simulink library "SUB_ECU_L4_MABX_HW_Interface_PTC_166"  (R2018a)
settings: Solver=VariableStepAuto  StartTime=0.0  StopTime=10.0  RelTol=1e-3
PostLoadFcn:
  | , if any(exist('dsrtsu_mdlpostloadfcn', 'file') == [2, 3, 6]), try dsrtsu_mdlpostloadfcn('Execute', bdroot); catch fprintf('Error in PostLoadFcn (dsrtsu_mdlpostloadfcn) for model "%s":\n %s\n', bdroot, lasterr); end, end,
undefined symbols (not defined in the file or in its folder): CANR_PROPB_REAX_3_13_CHANNEL_APV, CANR_PROPB_REAX_4_13_CHANNEL_APV, CANR_PROPB_XPR_1_50_CHANNEL_APV, ENUM_CAN_RX_T, ENUM_CAN_TX_T, ENUM_REAX_OPERATION_MODE_T, ENUM_SIGNAL_HEALTH_T, ENUM_XBR_CONTROL_MODE_T, ENUM_XBR_EBI_MODE_T, ENUM_XBR_PASS_THROUGH_ACTIVE_T, ENUM_XBR_PRIORITY_T, ENUM_XPR_INHIBIT_PARK_MANUAL_T, ENUM_XPR_INHIBIT_UNPARK_MANUAL_T, ENUM_XPR_PARK_MANUAL_T, ENUM_XPR_UNPARK_MANUAL_T, PROPB_REAX_1_E4_DES_POS_SIG_SRC_APV, PROPB_REAX_1_E4_DESIRED_OPMODE_APV, PROPB_REAX_1_E4_DESIRED_POSITION_APV, ptc_matlab_lib
libraries: PTC_MBDS_LIB x163, rtican x79, simulink x41, EmE_MBD_Blockset x35, rti1401lib_dio_type4 x8, simulink_need_slupdate x7, $bdroot x5, rti1401lib_adc_type4 x3, rtitasklib x1
(part 3 of 25)

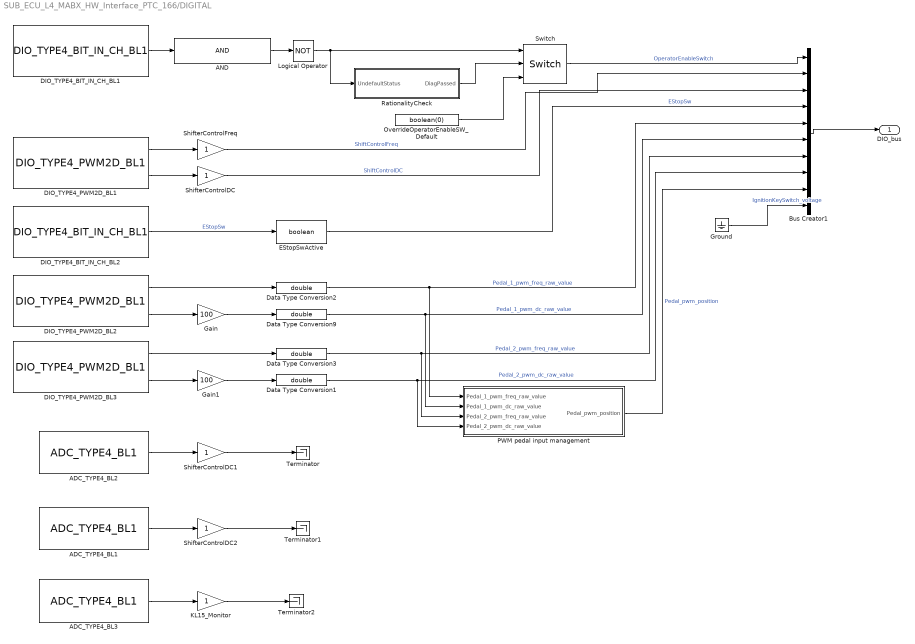
== system SUB_ECU_L4_MABX_HW_Interface_PTC_166/DIGITAL ==
  ADC_TYPE4_BL1 : rti1401lib_adc_type4/ADC_TYPE4_BL1  DSProperties=struct('RTI',struct('Version',uint32(2),'BlockType',struct('isSLSource',uint8(1),'isSLSink',uint8(1),'isHWSource',uint8(0),'isHWSink',uint8(1),'isSetup',uint8(0),'isInline',uint8(1),'isNonInline',uint8(0),'isInterrupt',uint8(0),'isChannelwise',uint8(1)),'IOBoardType',{{'DS1401','STD','ADCT4'}},'UnitType','ADC','Identifier','ADC','DialogType','ML','BlockSet','NONE','SlaveProcessor','NONE'))  RTIBlockInterface=struct('InputPortsActive',0,'InputPortsWidth',int32(1),'InputPortsDataType',{{'SS_BOOLEAN'}},'InputPortsName',{{'Continue'}},'OutputPortsActive',[1 0],'OutputPortsWidth',int32([1 1]),'OutputPortsDataType',{{'SS_DOUBLE','SS_UINT8'}},'OutputPortsName',{{'ADC','Status'}},'DialogFcn','rti1401stdadct4adcgui','SampleTime',{{-1}},'InitLevel',3,'IconTransparency','on','BlockDisplay',{{['ADC TP4\nModule: 1\nChannel: 2'],'center'}},'BlockName',struct('Token',{{'ADC_TYPE4_BL1'}}))  RTIBlockParameters=struct('ADCSWStartDisable',{{0,'OFF',[0 1]}},'ModuleNo',{{1,'OFF',[1 16]}},'ChannelNo',{{2,'OFF',[1 16]}},'ConversionMode',{{1,'OFF',[1 2]}},'SampleMode',{{1,'OFF',[1 2]}},'TriggerSource',{{1,'OFF',[1 5]}},'EdgePolarity',{{1,'OFF',[1 2]}},'ConversionTriggerSource',{{2,'OFF',[1 6]}},'ConversionEdgePolarity',{{1,'OFF',[1 2]}},'ConversionPeriod',{{'1e-06','OFF',[]}},'ConversionPeriodCheck',{{0,'OFF',[]}},'BurstTriggerSource',{{1,'OFF',[1 6]}},'BurstEdgePolarity',{{1,'OFF',[1 2]}},'BurstSize',{{'10','OFF',[]}},'BurstSizeCheck',{{0,'OFF',[]}},'DataSetOffset',{{'0','OFF',[]}},'DataSetOffsetCheck',{{0,'OFF',[]}},'DataSetLength',{{'1','OFF',[]}},'DataSetLengthCheck',{{0,'OFF',[]}},'ReadMode',{{1,'OFF',[1 2]}},'SampleTime',{{'-1','OFF',[-1 inf]}},'SampleTimeCheck',{{1,'OFF',[]}},'StatusPortEnable',{{0,'OFF',[0 1]}},'VoltageRange',{{2,'OFF',[1 2]}},'TLCFileName',{{'rti1401adc_t4_adc','OFF',[]}})  RTISFcnParameters=struct('ADCSWStartDisable','int32','ModuleNo','int32','ChannelNo','int16','ConversionMode','int16','SampleMode','int16','TriggerSource','int16','EdgePolarity','int16','ConversionTriggerSource','int16','ConversionEdgePolarity','int16','ConversionPeriod','double','BurstTriggerSource','int16','BurstEdgePolarity','int16','BurstSize','int16','DataSetOffset','int16','DataSetLength','int16','ReadMode','int16','SampleTime','double','StatusPortEnable','int16','VoltageRange','int16','TLCFileName','char')  RTIBlockParaDefault=struct('ADCSWStartDisable',0,'ModuleNo',1,'ChannelNo',1,'ConversionMode',1,'SampleMode',1,'TriggerSource',1,'EdgePolarity',1,'ConversionTriggerSource',2,'ConversionEdgePolarity',1,'ConversionPeriod',1e-6,'ConversionPeriodCheck',0,'BurstTriggerSource',1,'BurstEdgePolarity',1,'BurstSize',10,'BurstSizeCheck',0,'DataSetOffset',0,'DataSetOffsetCheck',0,'DataSetLength',1,'DataSetLengthCheck',0,'ReadMode',1,'SampleTime',-1,'SampleTimeCheck',1,'StatusPortEnable',0,'VoltageRange',1,'TLCFileName','rti1401adc_t4_adc')
  ADC_TYPE4_BL2 : rti1401lib_adc_type4/ADC_TYPE4_BL1  DSProperties=struct('RTI',struct('Version',uint32(2),'BlockType',struct('isSLSource',uint8(1),'isSLSink',uint8(1),'isHWSource',uint8(0),'isHWSink',uint8(1),'isSetup',uint8(0),'isInline',uint8(1),'isNonInline',uint8(0),'isInterrupt',uint8(0),'isChannelwise',uint8(1)),'IOBoardType',{{'DS1401','STD','ADCT4'}},'UnitType','ADC','Identifier','ADC','DialogType','ML','BlockSet','NONE','SlaveProcessor','NONE'))  RTIBlockInterface=struct('InputPortsActive',0,'InputPortsWidth',int32(1),'InputPortsDataType',{{'SS_BOOLEAN'}},'InputPortsName',{{'Continue'}},'OutputPortsActive',[1 0],'OutputPortsWidth',int32([1 1]),'OutputPortsDataType',{{'SS_DOUBLE','SS_UINT8'}},'OutputPortsName',{{'ADC','Status'}},'DialogFcn','rti1401stdadct4adcgui','SampleTime',{{-1}},'InitLevel',3,'IconTransparency','on','BlockDisplay',{{['ADC TP4\nModule: 1\nChannel: 1'],'center'}},'BlockName',struct('Token',{{'ADC_TYPE4_BL1'}}))  RTIBlockParameters=struct('ADCSWStartDisable',{{0,'OFF',[0 1]}},'ModuleNo',{{1,'OFF',[1 16]}},'ChannelNo',{{1,'OFF',[1 16]}},'ConversionMode',{{1,'OFF',[1 2]}},'SampleMode',{{1,'OFF',[1 2]}},'TriggerSource',{{1,'OFF',[1 5]}},'EdgePolarity',{{1,'OFF',[1 2]}},'ConversionTriggerSource',{{2,'OFF',[1 6]}},'ConversionEdgePolarity',{{1,'OFF',[1 2]}},'ConversionPeriod',{{'1e-06','OFF',[]}},'ConversionPeriodCheck',{{0,'OFF',[]}},'BurstTriggerSource',{{1,'OFF',[1 6]}},'BurstEdgePolarity',{{1,'OFF',[1 2]}},'BurstSize',{{'10','OFF',[]}},'BurstSizeCheck',{{0,'OFF',[]}},'DataSetOffset',{{'0','OFF',[]}},'DataSetOffsetCheck',{{0,'OFF',[]}},'DataSetLength',{{'1','OFF',[]}},'DataSetLengthCheck',{{0,'OFF',[]}},'ReadMode',{{1,'OFF',[1 2]}},'SampleTime',{{'-1','OFF',[-1 inf]}},'SampleTimeCheck',{{1,'OFF',[]}},'StatusPortEnable',{{0,'OFF',[0 1]}},'VoltageRange',{{2,'OFF',[1 2]}},'TLCFileName',{{'rti1401adc_t4_adc','OFF',[]}})  RTISFcnParameters=struct('ADCSWStartDisable','int32','ModuleNo','int32','ChannelNo','int16','ConversionMode','int16','SampleMode','int16','TriggerSource','int16','EdgePolarity','int16','ConversionTriggerSource','int16','ConversionEdgePolarity','int16','ConversionPeriod','double','BurstTriggerSource','int16','BurstEdgePolarity','int16','BurstSize','int16','DataSetOffset','int16','DataSetLength','int16','ReadMode','int16','SampleTime','double','StatusPortEnable','int16','VoltageRange','int16','TLCFileName','char')  RTIBlockParaDefault=struct('ADCSWStartDisable',0,'ModuleNo',1,'ChannelNo',1,'ConversionMode',1,'SampleMode',1,'TriggerSource',1,'EdgePolarity',1,'ConversionTriggerSource',2,'ConversionEdgePolarity',1,'ConversionPeriod',1e-6,'ConversionPeriodCheck',0,'BurstTriggerSource',1,'BurstEdgePolarity',1,'BurstSize',10,'BurstSizeCheck',0,'DataSetOffset',0,'DataSetOffsetCheck',0,'DataSetLength',1,'DataSetLengthCheck',0,'ReadMode',1,'SampleTime',-1,'SampleTimeCheck',1,'StatusPortEnable',0,'VoltageRange',1,'TLCFileName','rti1401adc_t4_adc')
  ADC_TYPE4_BL3 : rti1401lib_adc_type4/ADC_TYPE4_BL1  DSProperties=struct('RTI',struct('Version',uint32(2),'BlockType',struct('isSLSource',uint8(1),'isSLSink',uint8(1),'isHWSource',uint8(0),'isHWSink',uint8(1),'isSetup',uint8(0),'isInline',uint8(1),'isNonInline',uint8(0),'isInterrupt',uint8(0),'isChannelwise',uint8(1)),'IOBoardType',{{'DS1401','STD','ADCT4'}},'UnitType','ADC','Identifier','ADC','DialogType','ML','BlockSet','NONE','SlaveProcessor','NONE'))  RTIBlockInterface=struct('InputPortsActive',0,'InputPortsWidth',int32(1),'InputPortsDataType',{{'SS_BOOLEAN'}},'InputPortsName',{{'Continue'}},'OutputPortsActive',[1 0],'OutputPortsWidth',int32([1 1]),'OutputPortsDataType',{{'SS_DOUBLE','SS_UINT8'}},'OutputPortsName',{{'ADC','Status'}},'DialogFcn','rti1401stdadct4adcgui','SampleTime',{{-1}},'InitLevel',3,'IconTransparency','on','BlockDisplay',{{['ADC TP4\nModule: 1\nChannel: 3'],'center'}},'BlockName',struct('Token',{{'ADC_TYPE4_BL1'}}))  RTIBlockParameters=struct('ADCSWStartDisable',{{0,'OFF',[0 1]}},'ModuleNo',{{1,'OFF',[1 16]}},'ChannelNo',{{3,'OFF',[1 16]}},'ConversionMode',{{1,'OFF',[1 2]}},'SampleMode',{{1,'OFF',[1 2]}},'TriggerSource',{{1,'OFF',[1 5]}},'EdgePolarity',{{1,'OFF',[1 2]}},'ConversionTriggerSource',{{2,'OFF',[1 6]}},'ConversionEdgePolarity',{{1,'OFF',[1 2]}},'ConversionPeriod',{{'1e-06','OFF',[]}},'ConversionPeriodCheck',{{0,'OFF',[]}},'BurstTriggerSource',{{1,'OFF',[1 6]}},'BurstEdgePolarity',{{1,'OFF',[1 2]}},'BurstSize',{{'10','OFF',[]}},'BurstSizeCheck',{{0,'OFF',[]}},'DataSetOffset',{{'0','OFF',[]}},'DataSetOffsetCheck',{{0,'OFF',[]}},'DataSetLength',{{'1','OFF',[]}},'DataSetLengthCheck',{{0,'OFF',[]}},'ReadMode',{{1,'OFF',[1 2]}},'SampleTime',{{'-1','OFF',[-1 inf]}},'SampleTimeCheck',{{1,'OFF',[]}},'StatusPortEnable',{{0,'OFF',[0 1]}},'VoltageRange',{{2,'OFF',[1 2]}},'TLCFileName',{{'rti1401adc_t4_adc','OFF',[]}})  RTISFcnParameters=struct('ADCSWStartDisable','int32','ModuleNo','int32','ChannelNo','int16','ConversionMode','int16','SampleMode','int16','TriggerSource','int16','EdgePolarity','int16','ConversionTriggerSource','int16','ConversionEdgePolarity','int16','ConversionPeriod','double','BurstTriggerSource','int16','BurstEdgePolarity','int16','BurstSize','int16','DataSetOffset','int16','DataSetLength','int16','ReadMode','int16','SampleTime','double','StatusPortEnable','int16','VoltageRange','int16','TLCFileName','char')  RTIBlockParaDefault=struct('ADCSWStartDisable',0,'ModuleNo',1,'ChannelNo',1,'ConversionMode',1,'SampleMode',1,'TriggerSource',1,'EdgePolarity',1,'ConversionTriggerSource',2,'ConversionEdgePolarity',1,'ConversionPeriod',1e-6,'ConversionPeriodCheck',0,'BurstTriggerSource',1,'BurstEdgePolarity',1,'BurstSize',10,'BurstSizeCheck',0,'DataSetOffset',0,'DataSetOffsetCheck',0,'DataSetLength',1,'DataSetLengthCheck',0,'ReadMode',1,'SampleTime',-1,'SampleTimeCheck',1,'StatusPortEnable',0,'VoltageRange',1,'TLCFileName','rti1401adc_t4_adc')
  AND : PTC_MBDS_LIB/MBDS Standard Library/Basic Operations/Logic and Bit Operations/AND  BitwiseMode=on  Inputs=1  UseBitMask=on  BitMask=bin2dec('0000000000000001')  OutDataTypeStr=boolean  PTC_MBDS_BlockVersion=5.41  PTC_BlockType=PTC_MBDS_AND
      settings: AttributesFormatString=bitwise  SourceProductName=PACCAR Technical Center MBDS Library
  Bus Creator1 : BusCreator  Inputs=10
  DIO_TYPE4_BIT_IN_CH_BL1 : rti1401lib_dio_type4/DIO_TYPE4_BIT_IN_CH_BL1  DSProperties=struct('RTI',struct('Version',uint32(1),'BlockType',struct('isSLSource',uint8(1),'isSLSink',uint8(0),'isHWSource',uint8(1),'isHWSink',uint8(0),'isSetup',uint8(0),'isInline',uint8(1),'isNonInline',uint8(0),'isInterrupt',uint8(0),'isChannelwise',uint8(1)),'IOBoardType',{{'DS1401','STD','DIOT4'}},'UnitType','BIT','Identifier','BITINCH','DialogType','ML','BlockSet','NONE','SlaveProcessor','NONE'))  RTIBlockInterface=struct('OutputPortsWidth',int32(1),'OutputPortsDataType',{{'SS_BOOLEAN'}},'OutputPortsActive',1,'OutputPortsName',{{'Out'}},'BlockDisplay',{{['DIO TP4 BIT IN\n Channelwise\nModule: 1\nPort: 1\nChannel: 1'],'center'}},'IconTransparency','on','InitLevel',3,'DialogFcn','rti1401stddiot4bitinchgui','BlockName',struct('Token',{{'DIO_TYPE4_BIT_IN_CH_BL1'}}))  RTIBlockParameters=struct('ModuleNo',{{1,'OFF',[1 16]}},'PortNo',{{1,'OFF',[1 2]}},'ChannelNo',{{1,'OFF',[1 16]}},'TLCFileName',{{'rti1401dio_t4_bit_in_ch','OFF',[]}},'EnableInterrupt',{{0,'OFF',[0 1]}},'TriggerEdgeType',{{1,'OFF',[1 3]}})  RTISFcnParameters=struct('ModuleNo','int32','PortNo','int16','ChannelNo','int16','TLCFileName','char','EnableInterrupt','int16','TriggerEdgeType','int32')  RTIBlockParaDefault=struct('ModuleNo',1,'PortNo',1,'ChannelNo',1,'TLCFileName','rti1401dio_t4_bit_in_ch','EnableInterrupt',0,'TriggerEdgeType',1)
  DIO_TYPE4_BIT_IN_CH_BL2 : rti1401lib_dio_type4/DIO_TYPE4_BIT_IN_CH_BL1  DSProperties=struct('RTI',struct('Version',uint32(1),'BlockType',struct('isSLSource',uint8(1),'isSLSink',uint8(0),'isHWSource',uint8(1),'isHWSink',uint8(0),'isSetup',uint8(0),'isInline',uint8(1),'isNonInline',uint8(0),'isInterrupt',uint8(0),'isChannelwise',uint8(1)),'IOBoardType',{{'DS1401','STD','DIOT4'}},'UnitType','BIT','Identifier','BITINCH','DialogType','ML','BlockSet','NONE','SlaveProcessor','NONE'))  RTIBlockInterface=struct('OutputPortsWidth',int32(1),'OutputPortsDataType',{{'SS_BOOLEAN'}},'OutputPortsActive',1,'OutputPortsName',{{'Out'}},'BlockDisplay',{{['DIO TP4 BIT IN\n Channelwise\nModule: 1\nPort: 1\nChannel: 3'],'center'}},'IconTransparency','on','InitLevel',3,'DialogFcn','rti1401stddiot4bitinchgui','BlockName',struct('Token',{{'DIO_TYPE4_BIT_IN_CH_BL1'}}))  RTIBlockParameters=struct('ModuleNo',{{1,'OFF',[1 16]}},'PortNo',{{1,'OFF',[1 2]}},'ChannelNo',{{3,'OFF',[1 16]}},'TLCFileName',{{'rti1401dio_t4_bit_in_ch','OFF',[]}},'EnableInterrupt',{{0,'OFF',[0 1]}},'TriggerEdgeType',{{1,'OFF',[1 3]}})  RTISFcnParameters=struct('ModuleNo','int32','PortNo','int16','ChannelNo','int16','TLCFileName','char','EnableInterrupt','int16','TriggerEdgeType','int32')  RTIBlockParaDefault=struct('ModuleNo',1,'PortNo',1,'ChannelNo',1,'TLCFileName','rti1401dio_t4_bit_in_ch','EnableInterrupt',0,'TriggerEdgeType',1)
  DIO_TYPE4_PWM2D_BL1 : rti1401lib_dio_type4/DIO_TYPE4_PWM2D_BL1  DSProperties=struct('RTI',struct('Version',uint32(1),'BlockType',struct('isSLSource',uint8(1),'isSLSink',uint8(0),'isHWSource',uint8(1),'isHWSink',uint8(0),'isSetup',uint8(0),'isInline',uint8(1),'isNonInline',uint8(0),'isInterrupt',uint8(0),'isChannelwise',uint8(1)),'IOBoardType',{{'DS1401','STD','DIOT4'}},'UnitType','PWM','Identifier','PWM2D','DialogType','ML','BlockSet','NONE','SlaveProcessor','NONE'))  RTIBlockInterface=struct('OutputPortsWidth',int32([1 1]),'OutputPortsActive',[1 1],'OutputPortsName',{{'Frequency',['Duty Cycle']}},'BlockDisplay',{{['DIO TP4 PWM2D\nModule: 1\nPort: 1\nChannel: 2'],'center'}},'IconTransparency','on','InitLevel',3,'DialogFcn','rti1401stddiot4pwm2dgui','BlockName',struct('Token',{{'DIO_TYPE4_PWM2D_BL1'}}))  RTIBlockParameters=struct('ModuleNo',{{1,'ON',[1 16]}},'PortNo',{{1,'OFF',[1 2]}},'ChannelNo',{{2,'ON',[1 16]}},'UpdateMode',{{1,'ON',[1 2]}},'FrequencyRange',{{7,'OFF',[1 16]}},'TLCFileName',{{'rti1401dio_t4_pwm2d','OFF',[]}},'EnableInterrupt',{{0,'OFF',[0 1]}},'TriggerEdgeType',{{1,'OFF',[1 3]}})  RTISFcnParameters=struct('ModuleNo','int32','PortNo','int16','ChannelNo','int16','UpdateMode','int16','FrequencyRange','int16','TLCFileName','char','EnableInterrupt','int16','TriggerEdgeType','int32')  RTIBlockParaDefault=struct('ModuleNo',1,'PortNo',1,'ChannelNo',1,'UpdateMode',1,'FrequencyRange',7,'TLCFileName','rti1401dio_t4_pwm2d','EnableInterrupt',0,'TriggerEdgeType',1)
  DIO_TYPE4_PWM2D_BL2 : rti1401lib_dio_type4/DIO_TYPE4_PWM2D_BL1  DSProperties=struct('RTI',struct('Version',uint32(1),'BlockType',struct('isSLSource',uint8(1),'isSLSink',uint8(0),'isHWSource',uint8(1),'isHWSink',uint8(0),'isSetup',uint8(0),'isInline',uint8(1),'isNonInline',uint8(0),'isInterrupt',uint8(0),'isChannelwise',uint8(1)),'IOBoardType',{{'DS1401','STD','DIOT4'}},'UnitType','PWM','Identifier','PWM2D','DialogType','ML','BlockSet','NONE','SlaveProcessor','NONE'))  RTIBlockInterface=struct('OutputPortsWidth',int32([1 1]),'OutputPortsActive',[1 1],'OutputPortsName',{{'Frequency',['Duty Cycle']}},'BlockDisplay',{{['DIO TP4 PWM2D\nModule: 1\nPort: 2\nChannel: 1'],'center'}},'IconTransparency','on','InitLevel',3,'DialogFcn','rti1401stddiot4pwm2dgui','BlockName',struct('Token',{{'DIO_TYPE4_PWM2D_BL1'}}))  RTIBlockParameters=struct('ModuleNo',{{1,'ON',[1 16]}},'PortNo',{{2,'OFF',[1 2]}},'ChannelNo',{{1,'ON',[1 8]}},'UpdateMode',{{1,'ON',[1 2]}},'FrequencyRange',{{12,'OFF',[1 16]}},'TLCFileName',{{'rti1401dio_t4_pwm2d','OFF',[]}},'EnableInterrupt',{{0,'OFF',[0 1]}},'TriggerEdgeType',{{1,'OFF',[1 3]}})  RTISFcnParameters=struct('ModuleNo','int32','PortNo','int16','ChannelNo','int16','UpdateMode','int16','FrequencyRange','int16','TLCFileName','char','EnableInterrupt','int16','TriggerEdgeType','int32')  RTIBlockParaDefault=struct('ModuleNo',1,'PortNo',1,'ChannelNo',1,'UpdateMode',1,'FrequencyRange',7,'TLCFileName','rti1401dio_t4_pwm2d','EnableInterrupt',0,'TriggerEdgeType',1)
  DIO_TYPE4_PWM2D_BL3 : rti1401lib_dio_type4/DIO_TYPE4_PWM2D_BL1  DSProperties=struct('RTI',struct('Version',uint32(1),'BlockType',struct('isSLSource',uint8(1),'isSLSink',uint8(0),'isHWSource',uint8(1),'isHWSink',uint8(0),'isSetup',uint8(0),'isInline',uint8(1),'isNonInline',uint8(0),'isInterrupt',uint8(0),'isChannelwise',uint8(1)),'IOBoardType',{{'DS1401','STD','DIOT4'}},'UnitType','PWM','Identifier','PWM2D','DialogType','ML','BlockSet','NONE','SlaveProcessor','NONE'))  RTIBlockInterface=struct('OutputPortsWidth',int32([1 1]),'OutputPortsActive',[1 1],'OutputPortsName',{{'Frequency',['Duty Cycle']}},'BlockDisplay',{{['DIO TP4 PWM2D\nModule: 1\nPort: 2\nChannel: 2'],'center'}},'IconTransparency','on','InitLevel',3,'DialogFcn','rti1401stddiot4pwm2dgui','BlockName',struct('Token',{{'DIO_TYPE4_PWM2D_BL1'}}))  RTIBlockParameters=struct('ModuleNo',{{1,'ON',[1 16]}},'PortNo',{{2,'OFF',[1 2]}},'ChannelNo',{{2,'ON',[1 8]}},'UpdateMode',{{1,'ON',[1 2]}},'FrequencyRange',{{12,'OFF',[1 16]}},'TLCFileName',{{'rti1401dio_t4_pwm2d','OFF',[]}},'EnableInterrupt',{{0,'OFF',[0 1]}},'TriggerEdgeType',{{1,'OFF',[1 3]}})  RTISFcnParameters=struct('ModuleNo','int32','PortNo','int16','ChannelNo','int16','UpdateMode','int16','FrequencyRange','int16','TLCFileName','char','EnableInterrupt','int16','TriggerEdgeType','int32')  RTIBlockParaDefault=struct('ModuleNo',1,'PortNo',1,'ChannelNo',1,'UpdateMode',1,'FrequencyRange',7,'TLCFileName','rti1401dio_t4_pwm2d','EnableInterrupt',0,'TriggerEdgeType',1)
  Data Type Conversion{1..3,9} (4 alike) : DataTypeConversion  OutDataTypeStr=double  SaturateOnIntegerOverflow=on
  EStopSwActive : DataTypeConversion  OutDataTypeStr=boolean
  Gain : Gain  Gain=100
  Gain1 : Gain  Gain=100
  Ground : Ground
  KL15_Monitor : Gain
  Logical Operator : Logic  Operator=NOT  AllPortsSameDT=off  OutDataTypeStr=boolean
  OverrideOperatorEnableSW_Default : Constant  Value=boolean(0)
  PWM pedal input management : Subsystem
  RationalityCheck : Subsystem
  ShifterControlDC : Gain
  ShifterControlDC1 : Gain
  ShifterControlDC2 : Gain
  ShifterControlFreq : Gain
  Switch : PTC_MBDS_LIB/MBDS Standard Library/Signals & Systems/Signal Routing/Switch  OutDataTypeStr_=Inherit: Inherit via back propagation  SaturateOnIntegerOverflow_=on  InputSameDT_=on  PTC_MBDS_BlockVersion=5.41  PTC_BlockType=PTC_MBDS_Switch
      settings: SourceProductName=PACCAR Technical Center MBDS Library
  Terminator : Terminator
  Terminator1 : Terminator
  Terminator2 : Terminator
  DIO_bus : Outport
  wires:
  ShifterControlDC2/1 -> Terminator1/1
  ShifterControlDC1/1 -> Terminator/1
  ADC_TYPE4_BL2/1 -> ShifterControlDC1/1
  ADC_TYPE4_BL1/1 -> ShifterControlDC2/1
  Data Type Conversion1/1 -> PWM pedal input management/4(Pedal_2_pwm_dc_raw_value), Bus Creator1/8  "Pedal_2_pwm_dc_raw_value"
  Data Type Conversion3/1 -> PWM pedal input management/3(Pedal_2_pwm_freq_raw_value), Bus Creator1/7  "Pedal_2_pwm_freq_raw_value"
  Data Type Conversion9/1 -> PWM pedal input management/2(Pedal_1_pwm_dc_raw_value), Bus Creator1/6  "Pedal_1_pwm_dc_raw_value"
  Data Type Conversion2/1 -> PWM pedal input management/1(Pedal_1_pwm_freq_raw_value), Bus Creator1/5  "Pedal_1_pwm_freq_raw_value"
  PWM pedal input management/1(Pedal_pwm_position) -> Bus Creator1/9  "Pedal_pwm_position"
  Gain1/1 -> Data Type Conversion1/1
  Gain/1 -> Data Type Conversion9/1
  DIO_TYPE4_PWM2D_BL3/1 -> Data Type Conversion3/1
  DIO_TYPE4_PWM2D_BL2/1 -> Data Type Conversion2/1
  DIO_TYPE4_PWM2D_BL3/2 -> Gain1/1
  DIO_TYPE4_PWM2D_BL2/2 -> Gain/1
  DIO_TYPE4_BIT_IN_CH_BL1/1 -> AND/1
  Switch/1 -> Bus Creator1/1  "OperatorEnableSwitch"
  AND/1 -> Logical Operator/1
  DIO_TYPE4_PWM2D_BL1/1 -> ShifterControlFreq/1
  DIO_TYPE4_PWM2D_BL1/2 -> ShifterControlDC/1
  Bus Creator1/1 -> DIO_bus/1
  ShifterControlFreq/1 -> Bus Creator1/2  "ShiftControlFreq"
  ShifterControlDC/1 -> Bus Creator1/3  "ShiftControlDC"
  EStopSwActive/1 -> Bus Creator1/4  "EStopSw"
  Logical Operator/1 -> RationalityCheck/1(UndefaultStatus), Switch/1
  OverrideOperatorEnableSW_Default/1 -> Switch/3
  RationalityCheck/1(DiagPassed) -> Switch/2
  DIO_TYPE4_BIT_IN_CH_BL2/1 -> EStopSwActive/1  "EStopSw"
  ADC_TYPE4_BL3/1 -> KL15_Monitor/1
  KL15_Monitor/1 -> Terminator2/1
  Ground/1 -> Bus Creator1/10  "IgnitionKeySwitch_voltage"

== system SUB_ECU_L4_MABX_HW_Interface_PTC_166/DIGITAL_out ==
  Out : Inport
  In : Inport  Port=2
  Bus Selector : BusSelector  OutputSignals=10msTask.APTC.APTC_arb_pedal_position
  Constant1 : Constant
  Constant2 : Constant  Value=0.001
  Constant3 : Constant
  Constant4 : Constant  Value=0.001
  DIO_TYPE4_BIT_OUT_CH_BL1 : rti1401lib_dio_type4/DIO_TYPE4_BIT_OUT_CH_BL1  DSProperties=struct('RTI',struct('Version',uint32(1),'BlockType',struct('isSLSource',uint8(0),'isSLSink',uint8(1),'isHWSource',uint8(0),'isHWSink',uint8(1),'isSetup',uint8(0),'isInline',uint8(1),'isNonInline',uint8(0),'isInterrupt',uint8(0),'isChannelwise',uint8(1)),'IOBoardType',{{'DS1401','STD','DIOT4'}},'UnitType','BIT','Identifier','BITOUTCH','DialogType','ML','BlockSet','NONE','SlaveProcessor','NONE'))  RTIBlockInterface=struct('InputPortsWidth',int32(1),'InputPortsActive',1,'InputPortsDataType',{{'SS_BOOLEAN'}},'InputPortsName',{{'In'}},'BlockDisplay',{{['DIO TP4 BIT OUT\n Channelwise\nModule: 1\nPort: 1\nChannel: 3'],'center'}},'IconTransparency','on','InitLevel',3,'DialogFcn','rti1401stddiot4bitoutchgui','BlockName',struct('Token',{{'DIO_TYPE4_BIT_OUT_CH_BL1'}}))  RTIBlockParameters=struct('ModuleNo',{{1,'OFF',[1 16]}},'PortNo',{{1,'OFF',[1 2]}},'ChannelNo',{{3,'OFF',[1 16]}},'OutputStateInit',{{0,'OFF',[0 1]}},'TerminationMode',{{0,'OFF',[0 1]}},'OutputStateTermValidate',{{0,'OFF',[0 1]}},'OutputStateTerm',{{0,'OFF',[0 1]}},'SupplyRailsCh',{{[1 0],'OFF',[0 1 0 1]}},'TLCFileName',{{'rti1401dio_t4_bit_out_ch','OFF',[]}},'EnableInterrupt',{{0,'OFF',[0 1]}},'TriggerEdgeType',{{1,'OFF',[1 3]}})  RTISFcnParameters=struct('ModuleNo','int32','PortNo','int16','ChannelNo','int16','SupplyRailsCh','int16','OutputStateInit','int16','TerminationMode','int16','OutputStateTermValidate','int16','OutputStateTerm','int16','TLCFileName','char','EnableInterrupt','int16','TriggerEdgeType','int32')  RTIBlockParaDefault=struct('ModuleNo',1,'PortNo',1,'ChannelNo',1,'OutputStateInit',0,'TerminationMode',0,'OutputStateTermValidate',0,'OutputStateTerm',0,'SupplyRailsCh',[1 1],'TLCFileName','rti1401dio_t4_bit_out_ch','EnableInterrupt',0,'TriggerEdgeType',1)
  DIO_TYPE4_PWM_BL1 : rti1401lib_dio_type4/DIO_TYPE4_PWM_BL1  DSProperties=struct('RTI',struct('Version',uint32(1),'BlockType',struct('isSLSource',uint8(0),'isSLSink',uint8(1),'isHWSource',uint8(0),'isHWSink',uint8(1),'isSetup',uint8(0),'isInline',uint8(1),'isNonInline',uint8(0),'isInterrupt',uint8(0),'isChannelwise',uint8(1)),'IOBoardType',{{'DS1401','STD','DIOT4'}},'UnitType','PWM','Identifier','PWM','DialogType','ML','BlockSet','NONE','SlaveProcessor','NONE'))  RTIBlockInterface=struct('InputPortsWidth',int32([1 1]),'InputPortsActive',[1 1],'InputPortsName',{{'Period',['Duty Cycle']}},'BlockDisplay',{{['DIO TP4 PWM\nModule: 1\nPort: 2\nChannel: 1'],'center'}},'IconTransparency','on','InitLevel',3,'DialogFcn','rti1401stddiot4pwmgui','BlockName',struct('Token',{{'DIO_TYPE4_PWM_BL1'}}))  RTIBlockParameters=struct('ModuleNo',{{1,'OFF',[1 16]}},'PortNo',{{2,'OFF',[1 2]}},'ChannelNo',{{1,'OFF',[1 8]}},'SupplyRailsCh',{{[1 0],'OFF',[0 1 0 1]}},'UpdateMode',{{1,'ON',[1 2]}},'PeriodRange',{{2,'OFF',[1 16]}},'DutyCycleInit',{{'0.1','OFF',[0 1]}},'PeriodInit',{{'5e-03','OFF',[]}},'TerminationMode',{{0,'OFF',[0 1]}},'OutputTermValidate',{{0,'OFF',[0 1]}},'OutputTermBuildCheck',{{0,'OFF',[]}},'DutyCycleTerm',{{'0','OFF',[0 1]}},'PeriodTerm',{{'5e-05','OFF',[]}},'TLCFileName',{{'rti1401dio_t4_pwm','OFF',[]}},'EnableInterrupt',{{0,'OFF',[0 1]}},'TriggerEdgeType',{{1,'OFF',[1 3]}})  RTISFcnParameters=struct('ModuleNo','int32','PortNo','int16','ChannelNo','int16','SupplyRailsCh','int16','UpdateMode','int16','PeriodRange','int16','DutyCycleInit','double','PeriodInit','double','TerminationMode','int16','OutputTermValidate','int16','DutyCycleTerm','double','PeriodTerm','double','TLCFileName','char','EnableInterrupt','int16','TriggerEdgeType','int32')  RTIBlockParaDefault=struct('ModuleNo',1,'PortNo',1,'ChannelNo',1,'SupplyRailsCh',[1 1],'UpdateMode',1,'PeriodRange',7,'DutyCycleInit',0,'PeriodInit',5e-5,'TerminationMode',0,'OutputTermValidate',0,'OutputTermBuildCheck',0,'DutyCycleTerm',0,'PeriodTerm',5e-5,'TLCFileName','rti1401dio_t4_pwm','EnableInterrupt',0,'TriggerEdgeType',1)
  DIO_TYPE4_PWM_BL2 : rti1401lib_dio_type4/DIO_TYPE4_PWM_BL1  DSProperties=struct('RTI',struct('Version',uint32(1),'BlockType',struct('isSLSource',uint8(0),'isSLSink',uint8(1),'isHWSource',uint8(0),'isHWSink',uint8(1),'isSetup',uint8(0),'isInline',uint8(1),'isNonInline',uint8(0),'isInterrupt',uint8(0),'isChannelwise',uint8(1)),'IOBoardType',{{'DS1401','STD','DIOT4'}},'UnitType','PWM','Identifier','PWM','DialogType','ML','BlockSet','NONE','SlaveProcessor','NONE'))  RTIBlockInterface=struct('InputPortsWidth',int32([1 1]),'InputPortsActive',[1 1],'InputPortsName',{{'Period',['Duty Cycle']}},'BlockDisplay',{{['DIO TP4 PWM\nModule: 1\nPort: 2\nChannel: 2'],'center'}},'IconTransparency','on','InitLevel',3,'DialogFcn','rti1401stddiot4pwmgui','BlockName',struct('Token',{{'DIO_TYPE4_PWM_BL1'}}))  RTIBlockParameters=struct('ModuleNo',{{1,'OFF',[1 16]}},'PortNo',{{2,'OFF',[1 2]}},'ChannelNo',{{2,'OFF',[1 8]}},'SupplyRailsCh',{{[1 0],'OFF',[0 1 0 1]}},'UpdateMode',{{1,'ON',[1 2]}},'PeriodRange',{{2,'OFF',[1 16]}},'DutyCycleInit',{{'0.2','OFF',[0 1]}},'PeriodInit',{{'5e-03','OFF',[]}},'TerminationMode',{{0,'OFF',[0 1]}},'OutputTermValidate',{{0,'OFF',[0 1]}},'OutputTermBuildCheck',{{0,'OFF',[]}},'DutyCycleTerm',{{'0','OFF',[0 1]}},'PeriodTerm',{{'5e-05','OFF',[]}},'TLCFileName',{{'rti1401dio_t4_pwm','OFF',[]}},'EnableInterrupt',{{0,'OFF',[0 1]}},'TriggerEdgeType',{{1,'OFF',[1 3]}})  RTISFcnParameters=struct('ModuleNo','int32','PortNo','int16','ChannelNo','int16','SupplyRailsCh','int16','UpdateMode','int16','PeriodRange','int16','DutyCycleInit','double','PeriodInit','double','TerminationMode','int16','OutputTermValidate','int16','DutyCycleTerm','double','PeriodTerm','double','TLCFileName','char','EnableInterrupt','int16','TriggerEdgeType','int32')  RTIBlockParaDefault=struct('ModuleNo',1,'PortNo',1,'ChannelNo',1,'SupplyRailsCh',[1 1],'UpdateMode',1,'PeriodRange',7,'DutyCycleInit',0,'PeriodInit',5e-5,'TerminationMode',0,'OutputTermValidate',0,'OutputTermBuildCheck',0,'DutyCycleTerm',0,'PeriodTerm',5e-5,'TLCFileName','rti1401dio_t4_pwm','EnableInterrupt',0,'TriggerEdgeType',1)
  Data Type Conversion{1..2,5..6,9..10} (6 alike) : DataTypeConversion  OutDataTypeStr=double
  Determine pedal PWM and duty cycle values : Subsystem
  Divide : Product  Inputs=*/
  Divide1 : Product  Inputs=*/
  Gain : Gain  Gain=0.01
  Gain1 : Gain  Gain=0.01
  Logical Operator : Logic  Operator=NOT  AllPortsSameDT=off  OutDataTypeStr=boolean
  MinMax : MinMax  Function=max  Inputs=2  InputSameDT=on
  MinMax1 : MinMax  Function=max  Inputs=2  InputSameDT=on
  Shift Control : Subsystem
  wires:
  Determine pedal PWM and duty cycle values/3(APTC_PWM_pedalB_freq_out) -> MinMax1/1
  Determine pedal PWM and duty cycle values/1(APTC_PWM_pedalA_freq_out) -> MinMax/1
  MinMax/1 -> Data Type Conversion1/1
  MinMax1/1 -> Data Type Conversion2/1
  Constant4/1 -> MinMax1/2
  Constant2/1 -> MinMax/2
  Data Type Conversion10/1 -> DIO_TYPE4_PWM_BL2/2  "PWMOut_P2C2_DC"
  Data Type Conversion9/1 -> DIO_TYPE4_PWM_BL2/1  "PWMOut_P2C2_Period"
  Data Type Conversion6/1 -> DIO_TYPE4_PWM_BL1/2  "PWMOut_P2C1_DC"
  Data Type Conversion5/1 -> DIO_TYPE4_PWM_BL1/1  "PWMOut_P2C1_Period"
  Data Type Conversion2/1 -> Divide1/2
  Data Type Conversion1/1 -> Divide/2
  Gain1/1 -> Data Type Conversion6/1
  Gain/1 -> Data Type Conversion10/1
  Divide1/1 -> Data Type Conversion9/1
  Constant1/1 -> Divide1/1
  Divide/1 -> Data Type Conversion5/1
  Constant3/1 -> Divide/1
  Determine pedal PWM and duty cycle values/4(APTC_PWM_pedalB_DC_out) -> Gain/1
  Determine pedal PWM and duty cycle values/2(APTC_PWM_pedalA_DC_out) -> Gain1/1
  Out/1 -> Bus Selector/1
  Shift Control/1(Out) -> Logical Operator/1
  Logical Operator/1 -> DIO_TYPE4_BIT_OUT_CH_BL1/1
  In/1 -> Shift Control/1(In), Determine pedal PWM and duty cycle values/2(In)
  Bus Selector/1 -> Determine pedal PWM and duty cycle values/1(APTC_arb_pedal_position)  "<APTC_arb_pedal_position>"

== system SUB_ECU_L4_MABX_HW_Interface_PTC_166/ETHERNET ==
  Bus Creator1 : BusCreator  Inputs=4
  Ground{,1..3} (4 alike) : Ground
  for_logging : Gain
  for_logging1 : Gain
  m/s_2_kph : Gain  Gain=3.6
  m/s_2_kph1 : Gain  Gain=3.6
  PIC_Bus : Outport
  wires:
  Bus Creator1/1 -> PIC_Bus/1  "PIC_Bus"
  m/s_2_kph/1 -> Bus Creator1/3  "CurrentVelocity_kph"
  m/s_2_kph1/1 -> Bus Creator1/4  "TargetVelocity_kph"
  for_logging/1 -> Bus Creator1/1  "CurrentAzimuth_rad"
  for_logging1/1 -> Bus Creator1/2  "TargetAzimuth_rad"
  Ground3/1 -> m/s_2_kph1/1
  Ground2/1 -> m/s_2_kph/1
  Ground1/1 -> for_logging1/1
  Ground/1 -> for_logging/1

== system SUB_ECU_L4_MABX_HW_Interface_PTC_166/INPUTS_PTC_166 ==
  note: 2018120-JLe: Added for RobotWits Waypoints
  Bus Creator : BusCreator  Inputs=4
  CAN_Truck166 : $bdroot/CAN_Truck166
  DIGITAL : $bdroot/DIGITAL
  ETHERNET : $bdroot/ETHERNET
  Timer_Access : Subsystem
  Inputs : Outport
  wires:
  CAN_Truck166/1 -> Bus Creator/1  "CAN"
  Bus Creator/1 -> Inputs/1  "INPUTS"
  DIGITAL/1 -> Bus Creator/2  "DIO_Bus"
  Timer_Access/1(TimeStamp) -> CAN_Truck166/1, Bus Creator/3  "timeStamp"
  ETHERNET/1 -> Bus Creator/4

== system SUB_ECU_L4_MABX_HW_Interface_PTC_166/OUTPUTS_PTC_166 ==
  Outputs : Inport
  In : Inport  Port=2
  CAN_Out_PTC_166 : $bdroot/CAN_Out_PTC_166
  DIGITAL_out : $bdroot/DIGITAL_out
  wires:
  Outputs/1 -> DIGITAL_out/1, CAN_Out_PTC_166/1
  In/1 -> DIGITAL_out/2, CAN_Out_PTC_166/2

== system SUB_ECU_L4_MABX_HW_Interface_PTC_166/CAN_Out_PTC_166/CAN_TX_10000ms ==
  10000msCAN : Inport
  Terminator : Terminator
  wires:
  10000msCAN/1 -> Terminator/1

== system SUB_ECU_L4_MABX_HW_Interface_PTC_166/CAN_Out_PTC_166/CAN_TX_1000ms ==
  1000msCAN : Inport
  CAN_TX_AIR1_31 : Subsystem
  CAN_TX_AMB_00 : Subsystem
  Constant1 : Constant  Value=ENUM_CAN_TX_T.TX_CAN_4
  Constant2 : Constant  Value=ENUM_CAN_TX_T.TX_CAN_4
  wires:
  Constant1/1 -> CAN_TX_AMB_00/1(Channel)
  1000msCAN/1 -> CAN_TX_AIR1_31/2(Data), CAN_TX_AMB_00/2(Data)
  Constant2/1 -> CAN_TX_AIR1_31/1(Channel)

== system SUB_ECU_L4_MABX_HW_Interface_PTC_166/CAN_Out_PTC_166/CAN_TX_100ms ==
  100msCAN : Inport
  Feedthrough : Inport  Port=2
  Bus Selector : BusSelector  OutputSignals=INPUTS.DIO_Bus.OperatorEnableSwitch,INPUTS.CAN.VI_00.F_Truck166_VIN_Match
  Bus Selector1 : BusSelector  OutputSignals=INPUTS.DIO_Bus.OperatorEnableSwitch
  Bus Selector2 : BusSelector  OutputSignals=INPUTS.DIO_Bus.OperatorEnableSwitch,INPUTS.CAN.VI_00.F_Truck1571_VIN_Match
  CANT_PROPB_XPR_5B_CHANNEL_APV : Constant  Value=ENUM_CAN_TX_T.TX_CAN_1
  CANT_PROPB_XPR_FC_CHANNEL_APV : Constant  Value=ENUM_CAN_TX_T.TX_CAN_4
  CAN_TX_CCVS1_00 : Subsystem
  CAN_TX_PROPB_REAX_5_E4 : Subsystem
  CAN_TX_PROPB_XPR_5B : Subsystem
  CAN_TX_PROPB_XPR_FC : Subsystem
  COGSRapidUpdate : Subsystem
  EBC1_8B : Subsystem
  EffortsValue : Subsystem
  Encode_PropB_REAX_5 : Subsystem
  Encode_PropB_XPR_5B : Subsystem
  Encode_PropB_XPR_FC : Subsystem  SystemSampleTime=0.1
  Logical Operator : Logic  OutDataTypeStr=boolean
  Logical Operator1 : Logic  OutDataTypeStr=boolean
  POSRapidUpdate : Subsystem
  PROPB_XPR_INHIBIT_PARK_MANUAL_APV : Constant  Value=ENUM_XPR_INHIBIT_PARK_MANUAL_T.NO_OVERRIDE
  PROPB_XPR_INHIBIT_UNPARK_MANUAL_APV : Constant  Value=ENUM_XPR_INHIBIT_UNPARK_MANUAL_T.NO_OVERRIDE
  PROPB_XPR_PARK_MANUAL_APV : Constant  Value=ENUM_XPR_PARK_MANUAL_T.NO_OVERRIDE
  PROPB_XPR_UNPARK_MANUAL_APV : Constant  Value=ENUM_XPR_UNPARK_MANUAL_T.NO_OVERRIDE
  enableCOGSRapidUpdateTX : Constant  Value=boolean(1)
  enableEBC1_8B_TX : Constant  Value=boolean(1)
  enablePosRapidUpdateTX : Constant  Value=boolean(1)
  wires:
  Feedthrough/1 -> CAN_TX_CCVS1_00/1(Data), COGSRapidUpdate/2(Data), EBC1_8B/2(Data)
  Logical Operator1/1 -> CAN_TX_PROPB_XPR_FC/1(Enable)
  Bus Selector2/2 -> Logical Operator1/2  "<F_Truck1571_VIN_Match>"
  Bus Selector2/1 -> Logical Operator1/1  "<OperatorEnableSwitch>"
  Bus Selector/2 -> Logical Operator/2  "<F_Truck166_VIN_Match>"
  Logical Operator/1 -> CAN_TX_PROPB_XPR_5B/1(Enable)
  Bus Selector/1 -> Logical Operator/1  "<OperatorEnableSwitch>"
  Encode_PropB_XPR_5B/1(Data) -> CAN_TX_PROPB_XPR_5B/3(RawData)
  CANT_PROPB_XPR_5B_CHANNEL_APV/1 -> CAN_TX_PROPB_XPR_5B/2(Channel)
  enableEBC1_8B_TX/1 -> EBC1_8B/1(Enable)
  Encode_PropB_REAX_5/1(Data) -> CAN_TX_PROPB_REAX_5_E4/2(RawData)
  EffortsValue/1(EffortsValue) -> Encode_PropB_REAX_5/1(EffortsValue)
  Bus Selector1/1 -> Encode_PropB_XPR_FC/5(F_MessageEnable)  "<OperatorEnableSwitch>"
  CANT_PROPB_XPR_FC_CHANNEL_APV/1 -> CAN_TX_PROPB_XPR_FC/2(Channel)
  Encode_PropB_XPR_FC/1(Data) -> CAN_TX_PROPB_XPR_FC/3(RawData)
  PROPB_XPR_INHIBIT_UNPARK_MANUAL_APV/1 -> Encode_PropB_XPR_5B/2(inhibit_unpark_manual), Encode_PropB_XPR_FC/2(inhibit_unpark_manual)
  PROPB_XPR_PARK_MANUAL_APV/1 -> Encode_PropB_XPR_5B/3(park_manual), Encode_PropB_XPR_FC/3(park_manual)
  PROPB_XPR_UNPARK_MANUAL_APV/1 -> Encode_PropB_XPR_5B/4(unpark_manual), Encode_PropB_XPR_FC/4(unpark_manual)
  PROPB_XPR_INHIBIT_PARK_MANUAL_APV/1 -> Encode_PropB_XPR_5B/1(inhibit_park_manual), Encode_PropB_XPR_FC/1(inhibit_park_manual)
  enableCOGSRapidUpdateTX/1 -> COGSRapidUpdate/1(Enable)
  enablePosRapidUpdateTX/1 -> POSRapidUpdate/1(Enable)
  100msCAN/1 -> CAN_TX_PROPB_REAX_5_E4/1(enable), Bus Selector/1, Bus Selector1/1, POSRapidUpdate/2(Data), Bus Selector2/1

== system SUB_ECU_L4_MABX_HW_Interface_PTC_166/CAN_Out_PTC_166/CAN_TX_10ms ==
  10msCAN : Inport
  In : Inport  Port=2
  CANT_ACCS_E4_CHANNEL_APV : Constant  Value=ENUM_CAN_TX_T.TX_CAN_4
  CANT_EEC1_00_CHANNEL_APV : Constant  Value=ENUM_CAN_TX_T.TX_CAN_4_5
  CANT_VDC2_0B_CHANNEL_APV : Constant  Value=ENUM_CAN_TX_T.TX_CAN_5
  CAN_TX_ACCS_E4 : Subsystem
  CAN_TX_EEC1_00 : Subsystem
  CAN_TX_PROPB_REAX_1_E4 : Subsystem
  CAN_TX_VDC2_0B : Subsystem
  Encode_PROPB_REAX_1 : Subsystem
  wires:
  In/1 -> CAN_TX_EEC1_00/2(Data)
  CANT_ACCS_E4_CHANNEL_APV/1 -> CAN_TX_ACCS_E4/1(Channel)
  CANT_EEC1_00_CHANNEL_APV/1 -> CAN_TX_EEC1_00/1(Channel)
  Encode_PROPB_REAX_1/1(Out1) -> CAN_TX_PROPB_REAX_1_E4/2(RawData)
  CANT_VDC2_0B_CHANNEL_APV/1 -> CAN_TX_VDC2_0B/1(Channel)
  10msCAN/1 -> CAN_TX_PROPB_REAX_1_E4/1(enable), CAN_TX_VDC2_0B/2(Data), CAN_TX_ACCS_E4/2(Data), Encode_PROPB_REAX_1/1(In1)

== system SUB_ECU_L4_MABX_HW_Interface_PTC_166/CAN_Out_PTC_166/CAN_TX_20ms ==
  20msCAN : Inport
  Bus Selector : BusSelector  OutputSignals=INPUTS.DIO_Bus.OperatorEnableSwitch
  CANT_PROPB_XBR_B3_CHANNEL_APV : Constant  Value=ENUM_CAN_TX_T.TX_DISABLED
  CANT_STD_ODOMETRY_CHANNEL_APV : Constant  Value=ENUM_CAN_TX_T.TX_CAN_6
  CAN_TX_PROPB_XBR_B3 : Subsystem
  CAN_TX_PropB_2C2_XPR_65 : Subsystem
  CAN_TX_STD_ODOMETRY : Subsystem
  Encode_PropB_2C2_XPR : Subsystem
  Encode_PropB_XBR_B3 : Subsystem
  wires:
  Bus Selector/1 -> CAN_TX_PROPB_XBR_B3/3(OperatorEnable)  "<OperatorEnableSwitch>"
  Encode_PropB_XBR_B3/1(Out) -> CAN_TX_PROPB_XBR_B3/2(Data)
  CANT_PROPB_XBR_B3_CHANNEL_APV/1 -> CAN_TX_PROPB_XBR_B3/1(Channel)
  CANT_STD_ODOMETRY_CHANNEL_APV/1 -> CAN_TX_STD_ODOMETRY/1(Channel)
  20msCAN/1 -> CAN_TX_STD_ODOMETRY/2(Data), Encode_PropB_XBR_B3/1(In), Bus Selector/1, Encode_PropB_2C2_XPR/1(In)
  Encode_PropB_2C2_XPR/1(F_2C2_Enable) -> CAN_TX_PropB_2C2_XPR_65/1(Enable)
  Encode_PropB_2C2_XPR/2(Out) -> CAN_TX_PropB_2C2_XPR_65/2(RawData)

== system SUB_ECU_L4_MABX_HW_Interface_PTC_166/CAN_Out_PTC_166/CAN_TX_250ms ==
  250msCAN : Inport
  Terminator : Terminator
  wires:
  250msCAN/1 -> Terminator/1

== system SUB_ECU_L4_MABX_HW_Interface_PTC_166/CAN_Out_PTC_166/CAN_TX_5000ms ==
  5000msCAN : Inport
  Bus Selector : BusSelector  OutputSignals=INPUTS.DIO_Bus.OperatorEnableSwitch
  CAN_TX_RQST_13_E4 : Subsystem
  Encode_RQST : Subsystem
  RQST_13_E4_PGN : Subsystem
  wires:
  Bus Selector/1 -> CAN_TX_RQST_13_E4/2(OperatorEnable)  "<OperatorEnableSwitch>"
  5000msCAN/1 -> Bus Selector/1
  Encode_RQST/1(Data) -> CAN_TX_RQST_13_E4/1(RawData)
  RQST_13_E4_PGN/1(PGN) -> Encode_RQST/1(PGN)

== system SUB_ECU_L4_MABX_HW_Interface_PTC_166/CAN_Out_PTC_166/CAN_TX_50ms ==
  50msCAN : Inport
  CAN_TX_CCVS1 : Subsystem
  CAN_TX_TC1_05 : Subsystem
  enable_CAN_TX_CCVS1_CAN3 : Constant  OutDataTypeStr=Inherit: Inherit via back propagation
  wires:
  enable_CAN_TX_CCVS1_CAN3/1 -> CAN_TX_CCVS1/2(enable)
  50msCAN/1 -> CAN_TX_CCVS1/1(In1), CAN_TX_TC1_05/1(In1)

== system SUB_ECU_L4_MABX_HW_Interface_PTC_166/CAN_Out_PTC_166/CAN_TX_BAM ==
  CM : Subsystem
  Chart : Stateflow chart  TreatAsAtomicUnit=on
  Constant1 : Constant  Value=2  OutDataTypeStr=uint8
  DataFrame1 : Subsystem
  DataFrame2 : Subsystem
  Multiport Switch : MultiPortSwitch  Inputs=2  DiagnosticForDefault=Warning
  TX_TPCM : Subsystem
  TX_TPDT : Subsystem
  Terminator{,1..4} (5 alike) : Terminator
  Unit Delay1 : UnitDelay  InitialCondition=1  SampleTime=-1
  Unit Delay2 : UnitDelay  SampleTime=-1
  Unit Delay3 : UnitDelay  SampleTime=-1
  wires:
  Chart/5(TPDT_ts_Prev) -> Terminator4/1
  Chart/4(TPCM_ts_Prev) -> Terminator3/1
  Unit Delay1/1 -> Multiport Switch/1
  Unit Delay3/1 -> TX_TPDT/1(Trigger)
  Unit Delay2/1 -> TX_TPCM/1(Trigger)
  TX_TPDT/1(TX_status) -> Terminator1/1
  Chart/1(State) -> Terminator/1
  TX_TPCM/1(TX_status) -> Terminator2/1
  Chart/6(TPDT_count) -> Unit Delay1/1
  Chart/3(enTPCM) -> Unit Delay2/1
  Multiport Switch/1 -> TX_TPDT/2(Data)
  Constant1/1 -> Chart/3(TPDT_total)
  CM/1(Out1) -> TX_TPCM/2(Data)
  DataFrame2/1(Out1) -> Multiport Switch/3
  Chart/2(enTPDT) -> Unit Delay3/1
  DataFrame1/1(Out1) -> Multiport Switch/2
  TX_TPCM/2(TX_time) -> Chart/1(TPCM_ts)
  TX_TPDT/2(TX_time) -> Chart/2(TPDT_ts)

== system SUB_ECU_L4_MABX_HW_Interface_PTC_166/CAN_Out_PTC_166/CAN_TX_VariableRate ==
  Feedthrough : Inport
  CAN_TX_Std_SystemTime_01 : Subsystem
  wires:
  Feedthrough/1 -> CAN_TX_Std_SystemTime_01/1(Feedthrough)

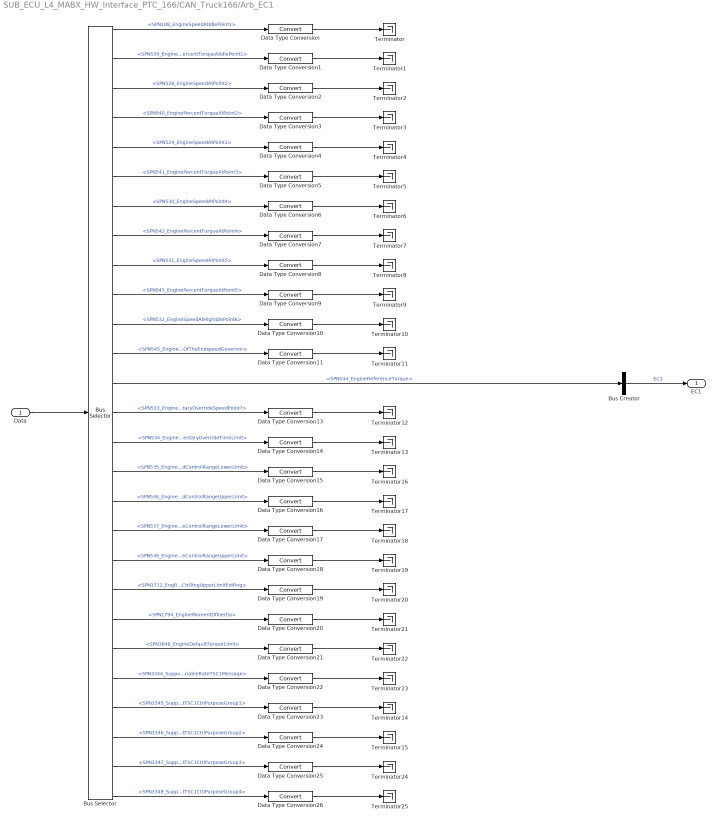
== system SUB_ECU_L4_MABX_HW_Interface_PTC_166/CAN_Truck166/Arb_EC1 ==
  Data : Inport
  Bus Creator : BusCreator  Inputs=1
  Bus Selector : BusSelector  OutputSignals=Signals.SPN188_EngineSpeedAtIdlePoint1,Signals.SPN539_EnginePercentTorqueAtIdlePoint1,Signals.SPN528_EngineSpeedAtPoint2,Signals.SPN540_EnginePercentTorqueAtPoint2,Signals.SPN529_EngineSpeedAtPoint3,Signals.SPN541_EnginePercentTorqueAtPoint3,Signals.SPN530_EngineSpeedAtPoint4,Signals.SPN542_EnginePercentTorqueAtPoint4,Signals.SPN531_EngineSpeedAtPoint5,Signals.SPN543_EnginePercentTorqueAtPoint5,Signals.SPN532_EngineSpeedAtHighIdlePoint6,Signals.SPN545_EngineGainKpOfTheEndspeedGovernor,Signals.SPN544_EngineReferenceTorque,Signals.SPN533_EngineMaximumMomentaryOverrideSpeedPoint7,Signals.SPN534_EngineMaximumMomentaryOverrideTimeLimit,Signals.SPN535_EngineRequestedSpeedControlRangeLowerLimit,Signals.SPN536_EngineRequestedSpeedControlRangeUpperLimit,Signals.SPN537_EngineRequestedTorqueControlRangeLowerLimit,Signals.SPN538_EngineRequestedTorqueControlRangeUpperLimit,Signals.SPN1712_EngRequestedSpeedCtrlRngUpperLimitExtRng,Signals.SPN1794_EngineMomentOfInertia,Signals.SPN1846_EngineDefaultTorqueLimit,Signals.SPN3344_SupportVariableRateTSC1Message,Signals.SPN3345_SupportTSC1CtrlPurposeGroup1,Signals.SPN3346_SupportTSC1CtrlPurposeGroup2,Signals.SPN3347_SupportTSC1CtrlPurposeGroup3,Signals.SPN3348_SupportTSC1CtrlPurposeGroup4
  Data Type Conversion{,1..11,13..26} (26 alike) : DataTypeConversion  SaturateOnIntegerOverflow=on
  Terminator{,1..25} (26 alike) : Terminator
      settings: InitFcn=|
      | try
      |    MBDS_BlockCallback('Update', gcb);
      | end
  EC1 : Outport
  wires:
  Bus Creator/1 -> EC1/1  "EC1"
  Data Type Conversion24/1 -> Terminator15/1
  Data Type Conversion25/1 -> Terminator24/1
  Data Type Conversion26/1 -> Terminator25/1
  Data Type Conversion19/1 -> Terminator20/1
  Data Type Conversion18/1 -> Terminator19/1
  Data Type Conversion21/1 -> Terminator22/1
  Data Type Conversion16/1 -> Terminator17/1
  Data Type Conversion17/1 -> Terminator18/1
  Data Type Conversion23/1 -> Terminator14/1
  Data Type Conversion22/1 -> Terminator23/1
  Data Type Conversion20/1 -> Terminator21/1
  Data Type Conversion11/1 -> Terminator11/1
  Data Type Conversion8/1 -> Terminator8/1
  Data Type Conversion15/1 -> Terminator16/1
  Data Type Conversion14/1 -> Terminator13/1
  Data Type Conversion13/1 -> Terminator12/1
  Data Type Conversion10/1 -> Terminator10/1
  Data Type Conversion9/1 -> Terminator9/1
  Data Type Conversion4/1 -> Terminator4/1
  Data Type Conversion7/1 -> Terminator7/1
  Data Type Conversion5/1 -> Terminator5/1
  Data Type Conversion6/1 -> Terminator6/1
  Data Type Conversion3/1 -> Terminator3/1
  Data Type Conversion2/1 -> Terminator2/1
  Data Type Conversion1/1 -> Terminator1/1
  Data Type Conversion/1 -> Terminator/1
  Bus Selector/27 -> Data Type Conversion26/1  "<SPN3348_SupportTSC1CtrlPurposeGroup4>"
  Bus Selector/26 -> Data Type Conversion25/1  "<SPN3347_SupportTSC1CtrlPurposeGroup3>"
  Bus Selector/25 -> Data Type Conversion24/1  "<SPN3346_SupportTSC1CtrlPurposeGroup2>"
  Bus Selector/24 -> Data Type Conversion23/1  "<SPN3345_SupportTSC1CtrlPurposeGroup1>"
  Bus Selector/23 -> Data Type Conversion22/1  "<SPN3344_SupportVariableRateTSC1Message>"
  Bus Selector/22 -> Data Type Conversion21/1  "<SPN1846_EngineDefaultTorqueLimit>"
  Bus Selector/21 -> Data Type Conversion20/1  "<SPN1794_EngineMomentOfInertia>"
  Bus Selector/20 -> Data Type Conversion19/1  "<SPN1712_EngRequestedSpeedCtrlRngUpperLimitExtRng>"
  Bus Selector/19 -> Data Type Conversion18/1  "<SPN538_EngineRequestedTorqueControlRangeUpperLimit>"
  Bus Selector/18 -> Data Type Conversion17/1  "<SPN537_EngineRequestedTorqueControlRangeLowerLimit>"
  Bus Selector/17 -> Data Type Conversion16/1  "<SPN536_EngineRequestedSpeedControlRangeUpperLimit>"
  Bus Selector/16 -> Data Type Conversion15/1  "<SPN535_EngineRequestedSpeedControlRangeLowerLimit>"
  Bus Selector/15 -> Data Type Conversion14/1  "<SPN534_EngineMaximumMomentaryOverrideTimeLimit>"
  Bus Selector/14 -> Data Type Conversion13/1  "<SPN533_EngineMaximumMomentaryOverrideSpeedPoint7>"
  Bus Selector/13 -> Bus Creator/1  "<SPN544_EngineReferenceTorque>"
  Bus Selector/11 -> Data Type Conversion10/1  "<SPN532_EngineSpeedAtHighIdlePoint6>"
  Bus Selector/10 -> Data Type Conversion9/1  "<SPN543_EnginePercentTorqueAtPoint5>"
  Bus Selector/9 -> Data Type Conversion8/1  "<SPN531_EngineSpeedAtPoint5>"
  Bus Selector/8 -> Data Type Conversion7/1  "<SPN542_EnginePercentTorqueAtPoint4>"
  Bus Selector/7 -> Data Type Conversion6/1  "<SPN530_EngineSpeedAtPoint4>"
  Bus Selector/6 -> Data Type Conversion5/1  "<SPN541_EnginePercentTorqueAtPoint3>"
  Bus Selector/5 -> Data Type Conversion4/1  "<SPN529_EngineSpeedAtPoint3>"
  Bus Selector/4 -> Data Type Conversion3/1  "<SPN540_EnginePercentTorqueAtPoint2>"
  Bus Selector/3 -> Data Type Conversion2/1  "<SPN528_EngineSpeedAtPoint2>"
  Bus Selector/2 -> Data Type Conversion1/1  "<SPN539_EnginePercentTorqueAtIdlePoint1>"
  Bus Selector/12 -> Data Type Conversion11/1  "<SPN545_EngineGainKpOfTheEndspeedGovernor>"
  Bus Selector/1 -> Data Type Conversion/1  "<SPN188_EngineSpeedAtIdlePoint1>"
  Data/1 -> Bus Selector/1

== system SUB_ECU_L4_MABX_HW_Interface_PTC_166/CAN_Truck166/Arb_PropB_REAX_3 ==
  Data : Inport
  Bus Selector : BusSelector  OutputSignals=Signals.PropB_REAX_3_CurrentOperatingMode,Signals.PropB_REAX_3_ReqOperatingMode,Signals.PropB_REAX_3_StatusErrMsg,Signals.PropB_REAX_3_HandwheelTorque,Signals.PropB_REAX_3_HandwheelVelocity,Signals.PropB_REAX_3_PullCompensation
  Data Type Conversion{,1..5} (6 alike) : DataTypeConversion  SaturateOnIntegerOverflow=on
  Terminator{,1..5} (6 alike) : Terminator
      settings: InitFcn=|
      | try
      |    MBDS_BlockCallback('Update', gcb);
      | end
  wires:
  Data Type Conversion5/1 -> Terminator5/1
  Data Type Conversion4/1 -> Terminator4/1
  Data Type Conversion3/1 -> Terminator3/1
  Data Type Conversion2/1 -> Terminator2/1
  Data Type Conversion1/1 -> Terminator1/1
  Data Type Conversion/1 -> Terminator/1
  Bus Selector/6 -> Data Type Conversion5/1  "<PropB_REAX_3_PullCompensation>"
  Bus Selector/5 -> Data Type Conversion4/1  "<PropB_REAX_3_HandwheelVelocity>"
  Bus Selector/1 -> Data Type Conversion/1  "<PropB_REAX_3_CurrentOperatingMode>"
  Bus Selector/3 -> Data Type Conversion2/1  "<PropB_REAX_3_StatusErrMsg>"
  Bus Selector/4 -> Data Type Conversion3/1  "<PropB_REAX_3_HandwheelTorque>"
  Bus Selector/2 -> Data Type Conversion1/1  "<PropB_REAX_3_ReqOperatingMode>"
  Data/1 -> Bus Selector/1

== system SUB_ECU_L4_MABX_HW_Interface_PTC_166/CAN_Truck166/Arb_PropB_REAX_4 ==
  Data : Inport
  Bus Selector : BusSelector  OutputSignals=Signals.PropB_REAX_4_AbsSteeringPosValid,Signals.PropB_REAX_4_PositionIndexValid,Signals.PropB_REAX_4_DriverControlledEffortsEnabled,Signals.PropB_REAX_4_ControlOperatingMode,Signals.PropB_REAX_4_SystemMode,Signals.PropB_REAX_4_PercHandwheelTorque,Signals.PropB_REAX_4_AbsSteeringAngle,Signals.PropB_REAX_4_PercMotorTorque
  Data Type Conversion{,1..7} (8 alike) : DataTypeConversion  SaturateOnIntegerOverflow=on
  Terminator{,1..7} (8 alike) : Terminator
      settings: InitFcn=|
      | try
      |    MBDS_BlockCallback('Update', gcb);
      | end
  wires:
  Data Type Conversion7/1 -> Terminator7/1
  Data Type Conversion6/1 -> Terminator6/1
  Data Type Conversion5/1 -> Terminator5/1
  Data Type Conversion4/1 -> Terminator4/1
  Data Type Conversion3/1 -> Terminator3/1
  Data Type Conversion2/1 -> Terminator2/1
  Data Type Conversion/1 -> Terminator1/1
  Data Type Conversion1/1 -> Terminator/1
  Bus Selector/8 -> Data Type Conversion7/1  "<PropB_REAX_4_PercMotorTorque>"
  Bus Selector/7 -> Data Type Conversion6/1  "<PropB_REAX_4_AbsSteeringAngle>"
  Bus Selector/6 -> Data Type Conversion5/1  "<PropB_REAX_4_PercHandwheelTorque>"
  Bus Selector/1 -> Data Type Conversion1/1  "<PropB_REAX_4_AbsSteeringPosValid>"
  Bus Selector/2 -> Data Type Conversion/1  "<PropB_REAX_4_PositionIndexValid>"
  Bus Selector/5 -> Data Type Conversion4/1  "<PropB_REAX_4_SystemMode>"
  Bus Selector/3 -> Data Type Conversion2/1  "<PropB_REAX_4_DriverControlledEffortsEnabled>"
  Bus Selector/4 -> Data Type Conversion3/1  "<PropB_REAX_4_ControlOperatingMode>"
  Data/1 -> Bus Selector/1

== system SUB_ECU_L4_MABX_HW_Interface_PTC_166/CAN_Truck166/CAN1_RX_TPCM_FF_00 ==
  Constant : Constant  Value=ENUM_CAN_RX_T.RX_CAN_1
  Multiport_Switch : MultiPortSwitch  DataPortOrder=Specify indices  DataPortIndices={ENUM_CAN_RX_T.RX_CAN_1, ENUM_CAN_RX_T.RX_CAN_2, ENUM_CAN_RX_T.RX_CAN_3, ENUM_CAN_RX_T.RX_CAN_4, ENUM_CAN_RX_T.RX_CAN_5, ENUM_CAN_RX_T.RX_CAN_6}  DataPortForDefault=Additional data port  SaturateOnIntegerOverflow=on  InputSameDT=on
      settings: AttributesFormatString=Zero-based indexing: %<zeroidx>
  RX_CAN_1 : Subsystem
  SelectChannel : Subsystem
  Terminator{,1..4} (5 alike) : Terminator
      settings: InitFcn=|
      | try
      |    MBDS_BlockCallback('Update', gcb);
      | end
  TPCM_FF_00 : Outport
  wires:
  Constant/1 -> SelectChannel/1(In1), Multiport_Switch/1
  SelectChannel/1(CAN1) -> RX_CAN_1/1(Enable)
  RX_CAN_1/1(TPCM_FF_00) -> Multiport_Switch/8, Multiport_Switch/7, Multiport_Switch/6, Multiport_Switch/5, Multiport_Switch/4, Multiport_Switch/3, Multiport_Switch/2
  SelectChannel/6(CAN6) -> Terminator4/1
  SelectChannel/5(CAN5) -> Terminator3/1
  SelectChannel/4(CAN4) -> Terminator2/1
  SelectChannel/3(CAN3) -> Terminator1/1
  SelectChannel/2(CAN2) -> Terminator/1
  Multiport_Switch/1 -> TPCM_FF_00/1

== system SUB_ECU_L4_MABX_HW_Interface_PTC_166/CAN_Truck166/CAN1_RX_TPDT_FF_00 ==
  Constant : Constant  Value=ENUM_CAN_RX_T.RX_CAN_1
  Multiport_Switch : MultiPortSwitch  DataPortOrder=Specify indices  DataPortIndices={ENUM_CAN_RX_T.RX_CAN_1, ENUM_CAN_RX_T.RX_CAN_2, ENUM_CAN_RX_T.RX_CAN_3, ENUM_CAN_RX_T.RX_CAN_4, ENUM_CAN_RX_T.RX_CAN_5, ENUM_CAN_RX_T.RX_CAN_6}  DataPortForDefault=Additional data port  SaturateOnIntegerOverflow=on  InputSameDT=on
      settings: AttributesFormatString=Zero-based indexing: %<zeroidx>
  RX_CAN_1 : Subsystem
  SelectChannel : Subsystem
  Terminator{,1..4} (5 alike) : Terminator
      settings: InitFcn=|
      | try
      |    MBDS_BlockCallback('Update', gcb);
      | end
  TPDT_FF_00 : Outport
  wires:
  Multiport_Switch/1 -> TPDT_FF_00/1
  SelectChannel/2(CAN2) -> Terminator/1
  SelectChannel/3(CAN3) -> Terminator1/1
  SelectChannel/4(CAN4) -> Terminator2/1
  SelectChannel/5(CAN5) -> Terminator3/1
  SelectChannel/6(CAN6) -> Terminator4/1
  RX_CAN_1/1(TPDT_FF_00) -> Multiport_Switch/2, Multiport_Switch/3, Multiport_Switch/4, Multiport_Switch/5, Multiport_Switch/6, Multiport_Switch/7, Multiport_Switch/8
  SelectChannel/1(CAN1) -> RX_CAN_1/1(Enable)
  Constant/1 -> Multiport_Switch/1, SelectChannel/1(In1)

== system SUB_ECU_L4_MABX_HW_Interface_PTC_166/CAN_Truck166/CAN_RX_ACC1_2A ==
  Constant : Constant  Value=boolean(1)
  RX_CAN_1 : Subsystem
  ACC1_2A : Outport
  wires:
  RX_CAN_1/1(ACC1_2A) -> ACC1_2A/1
  Constant/1 -> RX_CAN_1/1(Enable)

== system SUB_ECU_L4_MABX_HW_Interface_PTC_166/CAN_Truck166/CAN_RX_AEBS1_2A ==
  Constant : Constant  Value=boolean(1)
  RX_CAN_1 : Subsystem
  AEBS1_2A : Outport
  wires:
  Constant/1 -> RX_CAN_1/1(Enable)
  RX_CAN_1/1(AEBS1_2A) -> AEBS1_2A/1
